simulink model "power_PSTdeltahex"  (Simulink 6.0)
settings: Solver=ode23tb  StartTime=0.0  StopTime=50  MaxStep=1/60  RelTol=1e-4  AbsTol=1e-3
undefined symbols (not defined in the file or in its folder): I21_init_imag, I21_init_real
libraries: powerlib x117, powerlib_extras x19, simulink_extras x1
(part 2 of 3)

== system power_PSTdeltahex/Three-Phase OLTC Phase Shifting Transformer Delta-Hexagonal/TransfoB ==
  OLTC : Subsystem
  Transformer : Subsystem  AncestorBlock=powerlib/Elements/Multi-Winding Transformer  mask(Multi-Windings Transformer){LeftWindings=1, RightWindings=1, TappedWindings=taps on upper right winding, NumberOfTaps=19, NominalPower=[Pnom3ph/3 Fnom], NominalVoltages=Vnom_Windings, WindingResistances=Rpu_Windings, WindingInductances=Xpu_Windings, SetSaturation=off, Rm=Rmag, Lm=Lmag, Saturation=SaturationCurrentFlux, Hysteresis=off, DataFile='hysteresis.mat', Measurements=None, InitialFlux=26.7622502223547, TransfoNumber=1}
      mask prompts: LeftWindings "Number of windings on left side"; RightWindings "Number of windings on right side"; TappedWindings "Tapped winding"; NumberOfTaps "----  Number of taps (equally spaced):"; NominalPower "Nominal power and frequency [Pn(VA) fn(Hz)]:"; NominalVoltages "Winding nominal voltages [U1 U2 ... Un] (Vrms):"; WindingResistances "Winding resistances [R1 R2 ... Rn] (pu):"; WindingInductances "Winding leakage inductances [L1 L2 ... Ln] (pu):"; SetSaturation "Saturable core"; Rm "Magnetization resistance  Rm (pu)"; Lm "Magnetization reactance Lm (pu)"; Saturation "Saturation characteristic (pu) [ i1 ,  phi1 ;  i2 , phi2 ; ... ]"; Hysteresis "Simulate hysteresis"; DataFile "----  Hysteresis Data Mat file"; InitialFlux "Initial Flux (internal use)"; TransfoNumber "Device number (internal use)"
      mask init: same as power_PSTdeltahex/Three-Phase OLTC Phase Shifting Transformer Delta-Hexagonal/TransfoA/Transformer
      mask StyleString: edit,edit,popup(no taps|taps on upper left winding|taps on upper right winding),edit,edit,edit,edit,edit,checkbox,edit,edit,edit,checkbox,edit,popup(None|Winding voltages|Winding currents|Flux and excitation current ( Imag + IRm )|Flux and magnetization current ( Imag )|All measurements (V I Flux)),edit,edit
      mask CallbackString: powericon('NWindingsTransformerCback',gcb,0);|powericon('NWindingsTransformerCback',gcb,0);|powericon('NWindingsTransformerCback',gcb,1);|powericon('NWindingsTransformerCback',gcb,1);|||||powericon('NWindingsTransformerCback',gcb,0);||||powericon('NWindingsTransformerCback',gcb,0);||||
  W2- : PMIOPort  Orientation=left  Port=1  Side=Left
  W2_tap- : PMIOPort  Orientation=left  Port=2  Side=Left
  W1- : PMIOPort  Port=3  Side=Left
  W2+ : PMIOPort  Orientation=left  Port=4  Side=Right
  W2_tap+ : PMIOPort  Orientation=left  Port=5  Side=Right
  W1+ : PMIOPort  Port=6  Side=Right
  wires:
  [SwInversion] -> OLTC/3(SwInv)
  [SwTransfer] -> OLTC/2(SwR)
  [SwSelect] -> OLTC/1(Sw0/10)
  connections:
  W2-/RConn1 -- OLTC/LConn21 -- Transformer/RConn21
  Transformer/RConn20 -- OLTC/LConn20
  Transformer/RConn19 -- OLTC/LConn19
  Transformer/RConn18 -- OLTC/LConn18
  Transformer/RConn17 -- OLTC/LConn17
  Transformer/RConn16 -- OLTC/LConn16
  Transformer/RConn15 -- OLTC/LConn15
  Transformer/RConn14 -- OLTC/LConn14
  Transformer/RConn13 -- OLTC/LConn13
  Transformer/RConn12 -- OLTC/LConn12
  Transformer/RConn11 -- OLTC/LConn11
  Transformer/RConn10 -- OLTC/LConn10
  Transformer/RConn9 -- OLTC/LConn9
  Transformer/RConn8 -- OLTC/LConn8
  Transformer/RConn7 -- OLTC/LConn7
  Transformer/RConn6 -- OLTC/LConn6
  Transformer/RConn5 -- OLTC/LConn5
  Transformer/RConn4 -- OLTC/LConn4
  Transformer/RConn3 -- OLTC/LConn3
  Transformer/RConn2 -- OLTC/LConn2
  W2+/RConn1 -- OLTC/LConn1 -- Transformer/RConn1
  OLTC/RConn2 -- W2_tap-/RConn1
  OLTC/RConn1 -- W2_tap+/RConn1
  W1+/RConn1 -- Transformer/LConn1
  W1-/RConn1 -- Transformer/LConn2

== system power_PSTdeltahex/Three-Phase OLTC Phase Shifting Transformer Delta-Hexagonal/TransfoC ==
  OLTC : Subsystem
  Transformer : Subsystem  AncestorBlock=powerlib/Elements/Multi-Winding Transformer  mask(Multi-Windings Transformer){LeftWindings=1, RightWindings=1, TappedWindings=taps on upper right winding, NumberOfTaps=19, NominalPower=[Pnom3ph/3 Fnom], NominalVoltages=Vnom_Windings, WindingResistances=Rpu_Windings, WindingInductances=Xpu_Windings, SetSaturation=off, Rm=Rmag, Lm=Lmag, Saturation=SaturationCurrentFlux, Hysteresis=off, DataFile='hysteresis.mat', Measurements=None, InitialFlux=26.7622502223547, TransfoNumber=1}
      mask prompts: LeftWindings "Number of windings on left side"; RightWindings "Number of windings on right side"; TappedWindings "Tapped winding"; NumberOfTaps "----  Number of taps (equally spaced):"; NominalPower "Nominal power and frequency [Pn(VA) fn(Hz)]:"; NominalVoltages "Winding nominal voltages [U1 U2 ... Un] (Vrms):"; WindingResistances "Winding resistances [R1 R2 ... Rn] (pu):"; WindingInductances "Winding leakage inductances [L1 L2 ... Ln] (pu):"; SetSaturation "Saturable core"; Rm "Magnetization resistance  Rm (pu)"; Lm "Magnetization reactance Lm (pu)"; Saturation "Saturation characteristic (pu) [ i1 ,  phi1 ;  i2 , phi2 ; ... ]"; Hysteresis "Simulate hysteresis"; DataFile "----  Hysteresis Data Mat file"; InitialFlux "Initial Flux (internal use)"; TransfoNumber "Device number (internal use)"
      mask init: same as power_PSTdeltahex/Three-Phase OLTC Phase Shifting Transformer Delta-Hexagonal/TransfoA/Transformer
      mask StyleString: edit,edit,popup(no taps|taps on upper left winding|taps on upper right winding),edit,edit,edit,edit,edit,checkbox,edit,edit,edit,checkbox,edit,popup(None|Winding voltages|Winding currents|Flux and excitation current ( Imag + IRm )|Flux and magnetization current ( Imag )|All measurements (V I Flux)),edit,edit
      mask CallbackString: powericon('NWindingsTransformerCback',gcb,0);|powericon('NWindingsTransformerCback',gcb,0);|powericon('NWindingsTransformerCback',gcb,1);|powericon('NWindingsTransformerCback',gcb,1);|||||powericon('NWindingsTransformerCback',gcb,0);||||powericon('NWindingsTransformerCback',gcb,0);||||
  W2- : PMIOPort  Orientation=left  Port=1  Side=Left
  W2_tap- : PMIOPort  Orientation=left  Port=2  Side=Left
  W1- : PMIOPort  Port=3  Side=Left
  W2+ : PMIOPort  Orientation=left  Port=4  Side=Right
  W2_tap+ : PMIOPort  Orientation=left  Port=5  Side=Right
  W1+ : PMIOPort  Port=6  Side=Right
  wires:
  [SwSelect] -> OLTC/1(Sw0/10)
  [SwTransfer] -> OLTC/2(SwR)
  [SwInversion] -> OLTC/3(SwInv)
  connections:
  W1-/RConn1 -- Transformer/LConn2
  W1+/RConn1 -- Transformer/LConn1
  OLTC/RConn1 -- W2_tap+/RConn1
  OLTC/RConn2 -- W2_tap-/RConn1
  Transformer/RConn1 -- OLTC/LConn1 -- W2+/RConn1
  Transformer/RConn2 -- OLTC/LConn2
  Transformer/RConn3 -- OLTC/LConn3
  Transformer/RConn4 -- OLTC/LConn4
  Transformer/RConn5 -- OLTC/LConn5
  Transformer/RConn6 -- OLTC/LConn6
  Transformer/RConn7 -- OLTC/LConn7
  Transformer/RConn8 -- OLTC/LConn8
  Transformer/RConn9 -- OLTC/LConn9
  Transformer/RConn10 -- OLTC/LConn10
  Transformer/RConn11 -- OLTC/LConn11
  Transformer/RConn12 -- OLTC/LConn12
  Transformer/RConn13 -- OLTC/LConn13
  Transformer/RConn14 -- OLTC/LConn14
  Transformer/RConn15 -- OLTC/LConn15
  Transformer/RConn16 -- OLTC/LConn16
  Transformer/RConn17 -- OLTC/LConn17
  Transformer/RConn18 -- OLTC/LConn18
  Transformer/RConn19 -- OLTC/LConn19
  Transformer/RConn20 -- OLTC/LConn20
  Transformer/RConn21 -- OLTC/LConn21 -- W2-/RConn1

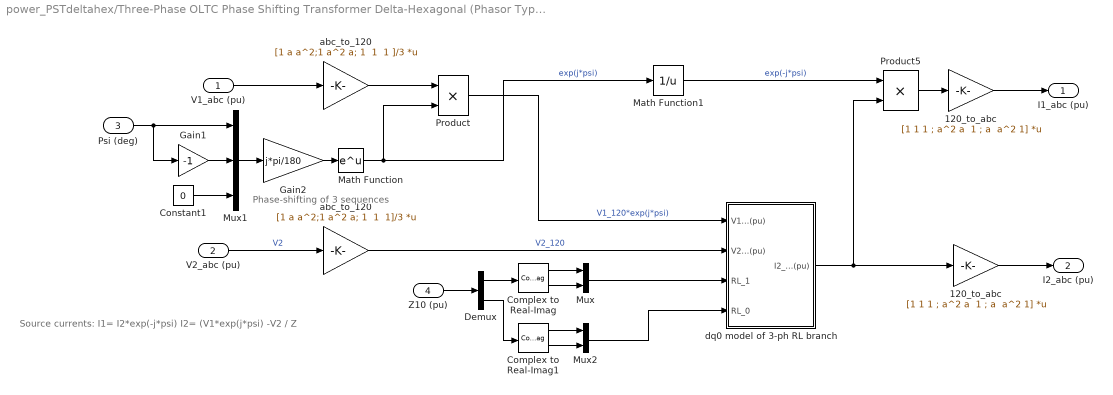
== system power_PSTdeltahex/Three-Phase OLTC Phase Shifting Transformer Delta-Hexagonal (Phasor Type)/ Currents ==
  note: Source currents:
      | I1= I2*exp(-j*psi)
      | I2= (V1*exp(j*psi) -V2 / Z
  note: Phase-shifting
      | of 3 sequences
  V1_abc (pu) : Inport  Port=1  LatchInput=off
  V2_abc (pu) : Inport  Port=2  LatchInput=off
  Psi (deg) : Inport  Port=3  LatchInput=off
  Z10 (pu) : Inport  Port=4  LatchInput=off
  120_to_abc : Gain  Gain="[1 1 1 ; a^2 a  1 ; a  a^2 1]"  Multiplication=Matrix(K*u)  SaturateOnIntegerOverflow=on
  "120_to_abc " : Gain  Gain="[1 1 1 ; a^2 a  1 ; a  a^2 1]"  Multiplication=Matrix(K*u)  SaturateOnIntegerOverflow=on
  Complex to Real-Imag : ComplexToRealImag
  Complex to Real-Imag1 : ComplexToRealImag
  Constant1 : Constant  Value=0
  Demux : Demux  Outputs=2
  Gain1 : Gain  Gain=-1  SaturateOnIntegerOverflow=on
  Gain2 : Gain  Gain=j*pi/180  SaturateOnIntegerOverflow=on
  Math Function : Math  SaturateOnIntegerOverflow=on
  Math Function1 : Math  Operator=reciprocal  SaturateOnIntegerOverflow=on
  Mux : Mux  Inputs=2
  Mux1 : Mux  Inputs=3
  Mux2 : Mux  Inputs=2
  Product : Product  SaturateOnIntegerOverflow=on
  Product5 : Product  SaturateOnIntegerOverflow=on
  abc_to_120 : Gain  Gain="[1 a a^2;1 a^2 a; 1  1  1 ]/3"  Multiplication=Matrix(K*u)  SaturateOnIntegerOverflow=on
  "abc_to_120 " : Gain  Gain="[1 a a^2;1 a^2 a; 1  1  1]/3"  Multiplication=Matrix(K*u)  SaturateOnIntegerOverflow=on
  dq0 model of 3-ph RL branch : Subsystem
  I1_abc (pu) : Outport
  "I2_abc (pu) " : Outport  Port=2
  wires:
  Gain2/1 -> Math Function/1
  Product/1 -> dq0 model of 3-ph RL branch/1(V1_120(pu))  "V1_120*exp(j*psi)"
  Math Function/1 -> Math Function1/1, Product/2  "exp(j*psi)"
  V1_abc (pu)/1 -> abc_to_120/1
  V2_abc (pu)/1 -> "abc_to_120 "/1  "V2"
  Product5/1 -> "120_to_abc "/1
  Z10 (pu)/1 -> Demux/1
  Math Function1/1 -> Product5/1  "exp(-j*psi)"
  Psi (deg)/1 -> Gain1/1, Mux1/1
  Mux1/1 -> Gain2/1
  Gain1/1 -> Mux1/2
  Constant1/1 -> Mux1/3
  dq0 model of 3-ph RL branch/1(I2_120 (pu)) -> Product5/2, 120_to_abc/1
  Demux/1 -> Complex to Real-Imag/1
  Demux/2 -> Complex to Real-Imag1/1
  Complex to Real-Imag/1 -> Mux/1
  Complex to Real-Imag/2 -> Mux/2
  Mux/1 -> dq0 model of 3-ph RL branch/3(RL_1)
  Complex to Real-Imag1/1 -> Mux2/1
  Complex to Real-Imag1/2 -> Mux2/2
  Mux2/1 -> dq0 model of 3-ph RL branch/4(RL_0)
  abc_to_120/1 -> Product/1
  "abc_to_120 "/1 -> dq0 model of 3-ph RL branch/2(V2_120(pu))  "V2_120"
  120_to_abc/1 -> "I2_abc (pu) "/1
  "120_to_abc "/1 -> I1_abc (pu)/1

== system power_PSTdeltahex/Three-Phase OLTC Phase Shifting Transformer Delta-Hexagonal (Phasor Type)/Current Source ==
  I1_abc : Inport  Orientation=left  Port=1  LatchInput=off
  I2_abc : Inport  Port=2  LatchInput=off
  Demux : Demux  Outputs=3
  Demux1 : Demux  Orientation=left  Outputs=3
  Gain2 : Gain  Gain=Ibase  SaturateOnIntegerOverflow=on
  Gain4 : Gain  Orientation=left  Gain=Ibase  SaturateOnIntegerOverflow=on
  Ground1 : powerlib/Elements/Ground  Orientation=down  PhysicalDomain=powersysdomain  SubClassName=unknown  LeftPortType=p1  RightPortType=p1  LConnTagsString=a
  Ground2 : powerlib/Elements/Ground  Orientation=down  PhysicalDomain=powersysdomain  SubClassName=unknown  LeftPortType=p1  RightPortType=p1  LConnTagsString=a
  IA : powerlib/Electrical Sources/Controlled Current Source  Initialize=on  Amplitude=I1A_init_mag  Phase=I1A_init_pha  Frequency=Fnom  Measurements=None
  IB : powerlib/Electrical Sources/Controlled Current Source  Initialize=on  Amplitude=I1B_init_mag  Phase=I1B_init_pha  Frequency=Fnom  Measurements=None
  IC : powerlib/Electrical Sources/Controlled Current Source  Initialize=on  Amplitude=I1C_init_mag  Phase=I1C_init_pha  Frequency=Fnom  Measurements=None
  Ia : powerlib/Electrical Sources/Controlled Current Source  Initialize=on  Amplitude=I2A_init_mag  Phase=I2A_init_pha  Frequency=Fnom  Measurements=None
  Ib : powerlib/Electrical Sources/Controlled Current Source  Initialize=on  Amplitude=I2B_init_mag  Phase=I2B_init_pha  Frequency=Fnom  Measurements=None
  Ic : powerlib/Electrical Sources/Controlled Current Source  Initialize=on  Amplitude=I2C_init_mag  Phase=I2C_init_pha  Frequency=Fnom  Measurements=None
  A : PMIOPort  Port=1  Side=Left
  a : PMIOPort  Orientation=left  Port=2  Side=Right
  B : PMIOPort  Port=3  Side=Left
  b : PMIOPort  Orientation=left  Port=4  Side=Right
  c : PMIOPort  Orientation=left  Port=5  Side=Right
  C : PMIOPort  Port=6  Side=Left
  wires:
  I1_abc/1 -> Gain4/1
  I2_abc/1 -> Gain2/1
  Demux/3 -> Ic/1
  Demux/2 -> Ib/1
  Demux/1 -> Ia/1
  Demux1/3 -> IC/1
  Demux1/2 -> IB/1
  Demux1/1 -> IA/1
  Gain2/1 -> Demux/1
  Gain4/1 -> Demux1/1
  connections:
  Ic/RConn1 -- c/RConn1
  Ib/RConn1 -- b/RConn1
  Ia/RConn1 -- a/RConn1
  C/RConn1 -- IC/LConn1
  B/RConn1 -- IB/LConn1
  A/RConn1 -- IA/LConn1
  Ib/LConn1 -- Ia/LConn1 -- Ic/LConn1 -- Ground1/LConn1
  IB/RConn1 -- IA/RConn1 -- IC/RConn1 -- Ground2/LConn1

== system power_PSTdeltahex/Three-Phase OLTC Phase Shifting Transformer Delta-Hexagonal (Phasor Type)/Subsystem ==
  note: Delta Hexagonal Phase Shifting Transformer
  note: Each phase consists of two windings ( winding W1(no taps)  and tapped winding W2)
      | Voltage ratio= 1:1  Rated voltage of each winding=2/3*(VnomPh-Ph)
      | Two OLTCs connected to inputs (ABC) and outputs (abc)
      | select taps symmetrical with respect to center of tapped windings W2
  note: A        a
      |                  |        |
      |              A A A A A A A A A A
      |            B          W2         C
      |          B                         C
      |        B    W1                  W1   C
      |      B                                 C
      |    B                                     C
      |  +                                         +
      |    C                                     B
      | c--->C                                 B<---B
      |        C    W2                  W2   B
      |     C--->C                         B<---b
      |            C          W1         B
      |              A A A A A A A A A A
  note: k=relative tap position
      |     k=Tap/NumberOfTaps  (-1<= k <= 1 )
      |
      | Psi= Phase shift  of output voltage (abc)  with respect to input voltage (ABC)
      | Psi varies from +60 deg. to -60 deg. when k varies from -1 to +1
      | Psi= 2*atan(-k/sqrt(3)
      |
      | Positive- and zero-sequence impedances vary with tap position k
  note: Positive sequence impedance:
      |  Z1 = Z1@ maximum_tap * kz1
      |           where :
      | kz1 =k/(2*(k^2+3))*(-3*k^2  +2k  +9)
      |   k  =  relative tap position (  0 <= k <=1 )
      |
      | Zero sequence impedance:
      |  Z0 = Zm*k^2

== system power_PSTdeltahex/Three-Phase OLTC Phase Shifting Transformer Delta-Hexagonal (Phasor Type)/Tap Changer Control ==
  Up : Inport  Port=1  LatchInput=off
  Down : Inport  Port=2  LatchInput=off
  Constant : Constant  Value=-1
  Constant1 : Constant
  Determine tap positon : Subsystem
  Edge Detector : powerlib_extras/Control  Blocks/Edge Detector  model=Rising  ic=0
  Logical Operator : Logic  Operator=OR  AllPortsSameDT=off
  Logical Operator1 : Logic  AllPortsSameDT=off
  Mechanical Delay : TransportDelay  DelayTime=MecDelay  InitialInput=InitialPosition
  Memory : Memory  Orientation=left  X0=1  InheritSampleTime=on
  Relational Operator : RelationalOperator  Operator===  LogicOutDataTypeMode=Specify via dialog  LogicDataType=float('double')
  Switch : Switch  Threshold=0.5  SaturateOnIntegerOverflow=on
  TapNo : Outport
  Ready : Outport  Port=2
  wires:
  Mechanical Delay/1 -> TapNo/1, Relational Operator/2
  Logical Operator1/1 -> Determine tap positon/Trigger
  Up/1 -> Logical Operator/1
  Down/1 -> Logical Operator/2, Switch/2
  Constant/1 -> Switch/1
  Constant1/1 -> Switch/3
  Switch/1 -> Determine tap positon/1(NewTap)
  Determine tap positon/1(TapNo) -> Mechanical Delay/1, Relational Operator/1
  Relational Operator/1 -> Memory/1
  Memory/1 -> Logical Operator1/1, Ready/1
  Logical Operator/1 -> Edge Detector/1
  Edge Detector/1 -> Logical Operator1/2

== system power_PSTdeltahex/Three-Phase OLTC Phase Shifting Transformer Delta-Hexagonal (Phasor Type)/Z1 Z0 impedances Computation  ==
  note: Positive sequence impedance:
      |  Z1 = Z1@ maximum_tap * kz1
      |           where :
      | kz1 =k/(2*(k^2+3))*(-3*k^2  +2k +9)
      |   k  =  relative tap position (  0 <= k <=1 )
      |
      | Zero sequence impedance:
      |  Z0 = Zm*k^2
  k : Inport  Port=1  LatchInput=off
  Z1maxpu : Inport  Port=2  LatchInput=off
  Zmpu : Inport  Port=3  LatchInput=off
  Abs : Abs  ZeroCross=off  SaturateOnIntegerOverflow=on
  Gain1 : Gain  Gain=2  SaturateOnIntegerOverflow=on
  Gain2 : Gain  Gain=3  SaturateOnIntegerOverflow=on
  Gain3 : Gain  Gain=2  SaturateOnIntegerOverflow=on
  Math Function2 : Math  Orientation=down  Operator=square  SaturateOnIntegerOverflow=on
  Mux : Mux  Inputs=2
  Product1 : Product  Inputs=*/*  SaturateOnIntegerOverflow=on
  Product5 : Product  Inputs=**  SaturateOnIntegerOverflow=on
  Product6 : Product  Inputs=**  SaturateOnIntegerOverflow=on
  Sum : Sum  SaturateOnIntegerOverflow=on
  Sum1 : Sum  Inputs=++-  SaturateOnIntegerOverflow=on
  psi4 : Constant  Value=3
  psi5 : Constant  Value=9
  Z10 : Outport
  wires:
  Product5/1 -> Mux/2  "Z0"
  Abs/1 -> Math Function2/1, Product1/1, Gain1/1  "k"
  k/1 -> Abs/1
  Mux/1 -> Z10/1
  Product6/1 -> Mux/1  "Z1"
  Product1/1 -> Product6/2  "kz1"
  Z1maxpu/1 -> Product6/1
  Zmpu/1 -> Product5/2
  Sum1/1 -> Product1/3  "-3*k^2 +2*k +9"
  psi5/1 -> Sum1/1
  psi4/1 -> Sum/2
  Sum/1 -> Gain3/1
  Math Function2/1 -> Sum/1, Product5/1, Gain2/1
  Gain1/1 -> Sum1/2
  Gain2/1 -> Sum1/3
  Gain3/1 -> Product1/2  "2*(k^2+3)"

== system power_PSTdeltahex/Three-Phase OLTC Phase Shifting Transformer Delta-Hexagonal (Phasor Type)/Zmin Saturation ==
  In1 : Inport  Port=1  LatchInput=off
  Complex to Real-Imag : ComplexToRealImag
  Real-Imag to Complex : RealImagToComplex
  Saturation2 : Saturate  UpperLimit=1000  LowerLimit=1e-3
  Saturation3 : Saturate  UpperLimit=1000  LowerLimit=1e-3
  Out1 : Outport
  wires:
  In1/1 -> Complex to Real-Imag/1
  Real-Imag to Complex/1 -> Out1/1
  Saturation3/1 -> Real-Imag to Complex/2
  Complex to Real-Imag/2 -> Saturation3/1
  Saturation2/1 -> Real-Imag to Complex/1
  Complex to Real-Imag/1 -> Saturation2/1

== system power_PSTdeltahex/Three-Phase OLTC Phase Shifting Transformer Delta-Hexagonal/OLTC Control/Monostable ==
  note: Monostable
  note: Silvano Casoria
      | Power System Simulation Laboratory
      | IREQ, Hydro-Quebec
  In : Inport  Port=1  LatchInput=off
  Clock : Clock
      settings: Decimation=10
  Edge Detector : Subsystem  mask(Edge Detector){model=EdgeDetect, ic=ic}
      mask prompts: model "Edge:"; ic "Input at t = -eps:"
      mask help:
      | This block compares its present input to its previous input.
      |
      | If the input  is a logic signal (TRUE (1) or FALSE (0), the output is a one-step boolean signal TRUE  when  the specified edge (Rising, Falling or Either)  is detected.
      |
      | This block can also be used to detect the slope polarity of a continuous signal. For example, if the specified edge is  "Rising", the output is TRUE as long as the slope of the input signal is positive.
      |
      | The input value at time preceeding t=0 is specified by the parameter "Input at t=-eps"
      mask init:
      | if model~=3,
      | 	x1 = (model -1)*20;
      |     x2 = (model -1)*60;
      | 	X1=[5,20,20,35]+25; Y1=[20+x2,20+x2,80-x2,80-x2];
      | 	X2=[5,20,35]+25;    Y2=[40+x1,60-x1,40+x1];
      | 	X3=[];X4=[];Y3=[];Y4=[];
      | else
      | 	x1 = 20;
      | 	x2 = 60;
      | 	X1=[5,20,20,35]+8; Y1=[20,20,80,80];
      | 	X2=[5,20,35]+8;    Y2=[40,60,40];
      | 	X3=[5,20,20,35]+53; Y3=[20+x2,20+x2,80-x2,80-x2];
      | 	X4=[5,20,35]+53;    Y4=[40+x1,60-x1,40+x1];
      | end
      mask Display: plot(0,0,100,100, X1,Y1,X2,Y2,X3,Y3,X4,Y4);
  Logical Operator1 : Logic
  Logical Operator2 : Logic  Orientation=left  Operator=NOT  Inputs=1
  Memory : Memory  Orientation=left  InheritSampleTime=on
  Relational Operator : RelationalOperator  Operator=>  InputSameDT=on
  Sample & Hold : powerlib_extras/Control  Blocks/Sample & Hold  ic=-1e6
  Sum : Sum  SaturateOnIntegerOverflow=on  InputSameDT=on
  T_monostable : Constant  Value=t_mono - eps
  Out : Outport
  wires:
  In/1 -> Edge Detector/1(In)
  Relational Operator/1 -> Out/1, Memory/1
  Logical Operator2/1 -> Logical Operator1/1
  Edge Detector/1(Out) -> Logical Operator1/2
  Memory/1 -> Logical Operator2/1
  Sample & Hold/1 -> Sum/1
  Sum/1 -> Relational Operator/1
  Clock/1 -> Relational Operator/2, Sample & Hold/1
  T_monostable/1 -> Sum/2
  Logical Operator1/1 -> Sample & Hold/2

== system power_PSTdeltahex/Three-Phase OLTC Phase Shifting Transformer Delta-Hexagonal/OLTC Control/Set Reset ==
  Tap : Inport  Port=1  LatchInput=off
  Constant1 : Constant  Value=-1
  Constant2 : Constant
  Edge Detector1 : powerlib_extras/Control  Blocks/Edge Detector  model=Rising  ic=0
  Edge Detector2 : powerlib_extras/Control  Blocks/Edge Detector  model=Falling  ic=0
  Logical Operator1 : Logic  AllPortsSameDT=off
  Logical Operator2 : Logic  AllPortsSameDT=off
  Relational Operator1 : RelationalOperator  Operator===
  Relational Operator2 : RelationalOperator  Operator===
  Set : Outport
  Reset : Outport  Port=2
  wires:
  Logical Operator1/1 -> Set/1
  Edge Detector1/1 -> Logical Operator1/1
  Relational Operator2/1 -> Logical Operator1/2
  Constant2/1 -> Relational Operator2/2
  Tap/1 -> Relational Operator2/1, Edge Detector1/1, Relational Operator1/1, Edge Detector2/1
  Logical Operator2/1 -> Reset/1
  Edge Detector2/1 -> Logical Operator2/1
  Relational Operator1/1 -> Logical Operator2/2
  Constant1/1 -> Relational Operator1/2

== system power_PSTdeltahex/Three-Phase OLTC Phase Shifting Transformer Delta-Hexagonal/OLTC Control/Tap Changer Control ==
  Up : Inport  Port=1  LatchInput=off
  Down : Inport  Port=2  LatchInput=off
  Constant : Constant  Value=-1
  Constant1 : Constant
  Determine tap positon : Subsystem
  Edge Detector : powerlib_extras/Control  Blocks/Edge Detector  model=Rising  ic=0
  Logical Operator : Logic  Operator=OR  AllPortsSameDT=off
  Logical Operator1 : Logic  AllPortsSameDT=off
  Mechanical Delay : TransportDelay  DelayTime=MecDelay  InitialInput=InitialPosition
  Memory : Memory  Orientation=left  X0=1  InheritSampleTime=on
  Relational Operator : RelationalOperator  Operator===  LogicOutDataTypeMode=Specify via dialog  LogicDataType=float('double')
  Switch : Switch  Threshold=0.5  SaturateOnIntegerOverflow=on
  TapNo : Outport
  Ready : Outport  Port=2
  wires:
  Edge Detector/1 -> Logical Operator1/2
  Logical Operator/1 -> Edge Detector/1
  Memory/1 -> Ready/1, Logical Operator1/1
  Relational Operator/1 -> Memory/1
  Determine tap positon/1(TapNo) -> Relational Operator/1, Mechanical Delay/1
  Switch/1 -> Determine tap positon/1(NewTap)
  Constant1/1 -> Switch/3
  Constant/1 -> Switch/1
  Down/1 -> Switch/2, Logical Operator/2
  Up/1 -> Logical Operator/1
  Logical Operator1/1 -> Determine tap positon/Trigger
  Mechanical Delay/1 -> Relational Operator/2, TapNo/1

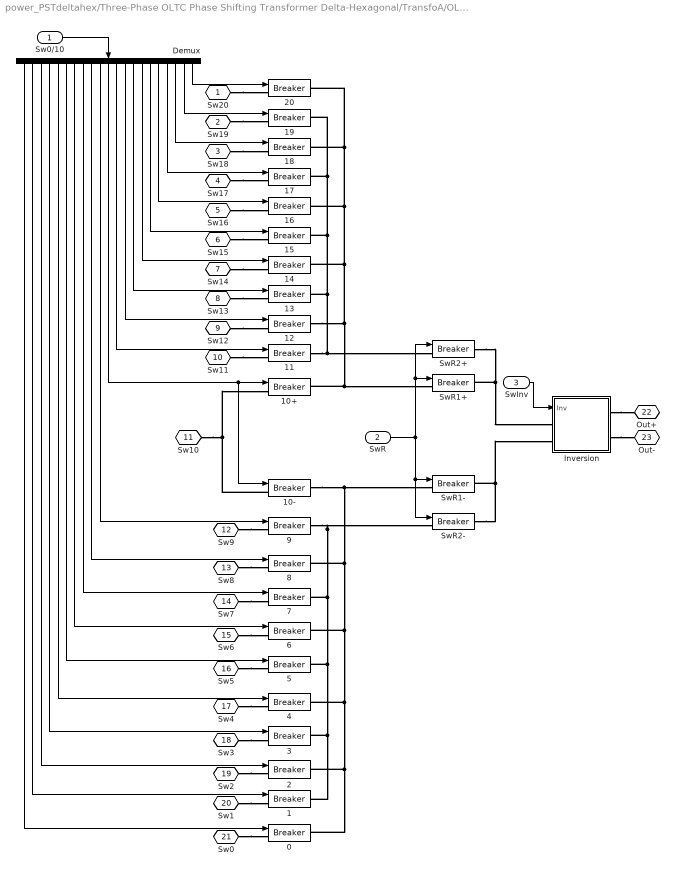
== system power_PSTdeltahex/Three-Phase OLTC Phase Shifting Transformer Delta-Hexagonal/TransfoA/OLTC ==
  Sw0/10 : Inport  Port=1  LatchInput=off
  SwR : Inport  Port=2  LatchInput=off
  SwInv : Inport  Port=3  LatchInput=off
  "0  " : powerlib/Elements/Breaker  BreakerResistance=Ron  InitialState=InitialStates(1)  SnubberResistance=Rsnub  SnubberCapacitance=inf  SwitchingTimes="[ 1/60  5/60 ]"  External=on  Measurements=None
  "1  " : powerlib/Elements/Breaker  BreakerResistance=Ron  InitialState=InitialStates(2)  SnubberResistance=Rsnub  SnubberCapacitance=inf  SwitchingTimes="[ 1/60  5/60 ]"  External=on  Measurements=None
  "10+  " : powerlib/Elements/Breaker  BreakerResistance=Ron  InitialState=InitialStates(11)  SnubberResistance=1e6  SnubberCapacitance=Rsnub  SwitchingTimes="[ 1/60  5/60 ]"  External=on  Measurements=None
  10- : powerlib/Elements/Breaker  BreakerResistance=Ron  InitialState=InitialStates(11)  SnubberResistance=Rsnub  SnubberCapacitance=inf  SwitchingTimes="[ 1/60  5/60 ]"  External=on  Measurements=None
  11 : powerlib/Elements/Breaker  BreakerResistance=Ron  InitialState=InitialStates(12)  SnubberResistance=Rsnub  SnubberCapacitance=inf  SwitchingTimes="[ 1/60  5/60 ]"  External=on  Measurements=None
  12 : powerlib/Elements/Breaker  BreakerResistance=Ron  InitialState=InitialStates(13)  SnubberResistance=Rsnub  SnubberCapacitance=inf  SwitchingTimes="[ 1/60  5/60 ]"  External=on  Measurements=None
  13 : powerlib/Elements/Breaker  BreakerResistance=Ron  InitialState=InitialStates(14)  SnubberResistance=Rsnub  SnubberCapacitance=inf  SwitchingTimes="[ 1/60  5/60 ]"  External=on  Measurements=None
  14 : powerlib/Elements/Breaker  BreakerResistance=Ron  InitialState=InitialStates(15)  SnubberResistance=Rsnub  SnubberCapacitance=inf  SwitchingTimes="[ 1/60  5/60 ]"  External=on  Measurements=None
  15 : powerlib/Elements/Breaker  BreakerResistance=Ron  InitialState=InitialStates(16)  SnubberResistance=Rsnub  SnubberCapacitance=inf  SwitchingTimes="[ 1/60  5/60 ]"  External=on  Measurements=None
  "16  " : powerlib/Elements/Breaker  BreakerResistance=Ron  InitialState=InitialStates(17)  SnubberResistance=Rsnub  SnubberCapacitance=inf  SwitchingTimes="[ 1/60  5/60 ]"  External=on  Measurements=None
  17 : powerlib/Elements/Breaker  BreakerResistance=Ron  InitialState=InitialStates(18)  SnubberResistance=Rsnub  SnubberCapacitance=inf  SwitchingTimes="[ 1/60  5/60 ]"  External=on  Measurements=None
  18 : powerlib/Elements/Breaker  BreakerResistance=Ron  InitialState=InitialStates(19)  SnubberResistance=Rsnub  SnubberCapacitance=inf  SwitchingTimes="[ 1/60  5/60 ]"  External=on  Measurements=None
  19 : powerlib/Elements/Breaker  BreakerResistance=Ron  InitialState=InitialStates(20)  SnubberResistance=Rsnub  SnubberCapacitance=inf  SwitchingTimes="[ 1/60  5/60 ]"  External=on  Measurements=None
  "2    " : powerlib/Elements/Breaker  BreakerResistance=Ron  InitialState=InitialStates(3)  SnubberResistance=Rsnub  SnubberCapacitance=inf  SwitchingTimes="[ 1/60  5/60 ]"  External=on  Measurements=None
  20 : powerlib/Elements/Breaker  BreakerResistance=Ron  InitialState=InitialStates(21)  SnubberResistance=Rsnub  SnubberCapacitance=inf  SwitchingTimes="[ 1/60  5/60 ]"  External=on  Measurements=None
  "3  " : powerlib/Elements/Breaker  BreakerResistance=Ron  InitialState=InitialStates(4)  SnubberResistance=Rsnub  SnubberCapacitance=inf  SwitchingTimes="[ 1/60  5/60 ]"  External=on  Measurements=None
  "4  " : powerlib/Elements/Breaker  BreakerResistance=Ron  InitialState=InitialStates(5)  SnubberResistance=Rsnub  SnubberCapacitance=inf  SwitchingTimes="[ 1/60  5/60 ]"  External=on  Measurements=None
  5 : powerlib/Elements/Breaker  BreakerResistance=Ron  InitialState=InitialStates(6)  SnubberResistance=Rsnub  SnubberCapacitance=inf  SwitchingTimes="[ 1/60  5/60 ]"  External=on  Measurements=None
  6 : powerlib/Elements/Breaker  BreakerResistance=Ron  InitialState=InitialStates(7)  SnubberResistance=Rsnub  SnubberCapacitance=inf  SwitchingTimes="[ 1/60  5/60 ]"  External=on  Measurements=None
  7 : powerlib/Elements/Breaker  BreakerResistance=Ron  InitialState=InitialStates(8)  SnubberResistance=Rsnub  SnubberCapacitance=inf  SwitchingTimes="[ 1/60  5/60 ]"  External=on  Measurements=None
  8 : powerlib/Elements/Breaker  BreakerResistance=Ron  InitialState=InitialStates(9)  SnubberResistance=Rsnub  SnubberCapacitance=inf  SwitchingTimes="[ 1/60  5/60 ]"  External=on  Measurements=None
  9 : powerlib/Elements/Breaker  BreakerResistance=Ron  InitialState=InitialStates(10)  SnubberResistance=Rsnub  SnubberCapacitance=inf  SwitchingTimes="[ 1/60  5/60 ]"  External=on  Measurements=None
  Demux : Demux  Orientation=down  Outputs=21
  Inversion : Subsystem
  SwR1+ : powerlib/Elements/Breaker  BreakerResistance=Ron  InitialState=1  SnubberResistance=R  SnubberCapacitance=inf  SwitchingTimes="[ 1/60  5/60 ]"  External=on  Measurements=None
  SwR1- : powerlib/Elements/Breaker  BreakerResistance=Ron  InitialState=1  SnubberResistance=R  SnubberCapacitance=inf  SwitchingTimes="[ 1/60  5/60 ]"  External=on  Measurements=None
  SwR2+ : powerlib/Elements/Breaker  BreakerResistance=Ron  InitialState=1  SnubberResistance=R  SnubberCapacitance=inf  SwitchingTimes="[ 1/60  5/60 ]"  External=on  Measurements=None
  SwR2- : powerlib/Elements/Breaker  BreakerResistance=Ron  InitialState=1  SnubberResistance=R  SnubberCapacitance=inf  SwitchingTimes="[ 1/60  5/60 ]"  External=on  Measurements=None
  Sw20 : PMIOPort  Port=1  Side=Left
  Sw19 : PMIOPort  Port=2  Side=Left
  Sw18 : PMIOPort  Port=3  Side=Left
  Sw17 : PMIOPort  Port=4  Side=Left
  Sw16 : PMIOPort  Port=5  Side=Left
  Sw15 : PMIOPort  Port=6  Side=Left
  Sw14 : PMIOPort  Port=7  Side=Left
  Sw13 : PMIOPort  Port=8  Side=Left
  Sw12 : PMIOPort  Port=9  Side=Left
  Sw11 : PMIOPort  Port=10  Side=Left
  Sw10 : PMIOPort  Port=11  Side=Left
  "Sw9 " : PMIOPort  Port=12  Side=Left
  Sw8 : PMIOPort  Port=13  Side=Left
  Sw7 : PMIOPort  Port=14  Side=Left
  Sw6 : PMIOPort  Port=15  Side=Left
  Sw5 : PMIOPort  Port=16  Side=Left
  Sw4 : PMIOPort  Port=17  Side=Left
  Sw3 : PMIOPort  Port=18  Side=Left
  "Sw2 " : PMIOPort  Port=19  Side=Left
  Sw1 : PMIOPort  Port=20  Side=Left
  Sw0 : PMIOPort  Port=21  Side=Left
  Out+ : PMIOPort  Orientation=left  Port=22  Side=Right
  Out- : PMIOPort  Orientation=left  Port=23  Side=Right
  wires:
  Sw0/10/1 -> Demux/1
  Demux/1 -> "0  "/1
  Demux/2 -> "1  "/1
  Demux/3 -> "2    "/1
  Demux/4 -> "3  "/1
  Demux/5 -> "4  "/1
  SwInv/1 -> Inversion/1(Inv)
  Demux/21 -> 20/1
  Demux/20 -> 19/1
  Demux/19 -> 18/1
  Demux/18 -> 17/1
  Demux/17 -> "16  "/1
  Demux/16 -> 15/1
  Demux/15 -> 14/1
  Demux/14 -> 13/1
  Demux/13 -> 12/1
  Demux/12 -> 11/1
  Demux/11 -> "10+  "/1, 10-/1
  Demux/10 -> 9/1
  Demux/9 -> 8/1
  Demux/8 -> 7/1
  Demux/7 -> 6/1
  Demux/6 -> 5/1
  SwR/1 -> SwR2+/1, SwR1+/1, SwR1-/1, SwR2-/1
  connections:
  Sw20/RConn1 -- 20/LConn1
  Sw19/RConn1 -- 19/LConn1
  Sw18/RConn1 -- 18/LConn1
  Sw17/RConn1 -- 17/LConn1
  Sw16/RConn1 -- "16  "/LConn1
  Sw4/RConn1 -- "4  "/LConn1
  Sw3/RConn1 -- "3  "/LConn1
  "Sw2 "/RConn1 -- "2    "/LConn1
  Sw1/RConn1 -- "1  "/LConn1
  Sw0/RConn1 -- "0  "/LConn1
  Inversion/RConn1 -- Out+/RConn1
  Inversion/RConn2 -- Out-/RConn1
  Sw5/RConn1 -- 5/LConn1
  Sw6/RConn1 -- 6/LConn1
  Sw7/RConn1 -- 7/LConn1
  Sw8/RConn1 -- 8/LConn1
  "Sw9 "/RConn1 -- 9/LConn1
  Sw15/RConn1 -- 15/LConn1
  Sw14/RConn1 -- 14/LConn1
  Sw13/RConn1 -- 13/LConn1
  Sw12/RConn1 -- 12/LConn1
  Sw11/RConn1 -- 11/LConn1
  SwR2-/RConn1 -- SwR1-/RConn1 -- Inversion/LConn2
  10-/RConn1 -- 8/RConn1 -- 6/RConn1 -- "4  "/RConn1 -- "2    "/RConn1 -- "0  "/RConn1 -- SwR1-/LConn1
  9/RConn1 -- 7/RConn1 -- 5/RConn1 -- "3  "/RConn1 -- "1  "/RConn1 -- SwR2-/LConn1
  12/RConn1 -- 14/RConn1 -- "16  "/RConn1 -- 18/RConn1 -- 20/RConn1 -- "10+  "/RConn1 -- SwR1+/LConn1
  11/RConn1 -- 13/RConn1 -- 15/RConn1 -- 17/RConn1 -- 19/RConn1 -- SwR2+/LConn1
  10-/LConn1 -- "10+  "/LConn1 -- Sw10/RConn1
  SwR2+/RConn1 -- SwR1+/RConn1 -- Inversion/LConn1

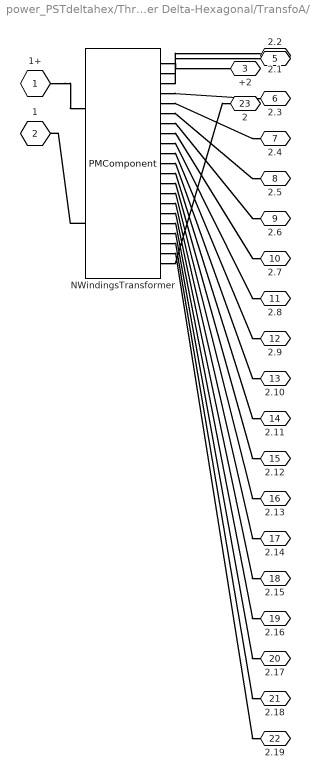
== system power_PSTdeltahex/Three-Phase OLTC Phase Shifting Transformer Delta-Hexagonal/TransfoA/Transformer ==
  NWindingsTransformer : PMComponent  PhysicalDomain=powersysdomain  LeftPortType=p1  RightPortType=p1  LConnTagsString=1|2  RConnTagsString=1|2|3|4|5|6|7|8|9|10|11|12|13|14|15|16|17|18|19|20|21
      mask Type: InnerPowersysBlock
  1+ : PMIOPort  Port=1  Side=Left
  1 : PMIOPort  Port=2  Side=Left
  +2 : PMIOPort  Orientation=left  Port=3  Side=Right
  2.1 : PMIOPort  Orientation=left  Port=4  Side=Right
  2.2 : PMIOPort  Orientation=left  Port=5  Side=Right
  2.3 : PMIOPort  Orientation=left  Port=6  Side=Right
  2.4 : PMIOPort  Orientation=left  Port=7  Side=Right
  2.5 : PMIOPort  Orientation=left  Port=8  Side=Right
  2.6 : PMIOPort  Orientation=left  Port=9  Side=Right
  2.7 : PMIOPort  Orientation=left  Port=10  Side=Right
  2.8 : PMIOPort  Orientation=left  Port=11  Side=Right
  2.9 : PMIOPort  Orientation=left  Port=12  Side=Right
  2.10 : PMIOPort  Orientation=left  Port=13  Side=Right
  2.11 : PMIOPort  Orientation=left  Port=14  Side=Right
  2.12 : PMIOPort  Orientation=left  Port=15  Side=Right
  2.13 : PMIOPort  Orientation=left  Port=16  Side=Right
  2.14 : PMIOPort  Orientation=left  Port=17  Side=Right
  2.15 : PMIOPort  Orientation=left  Port=18  Side=Right
  2.16 : PMIOPort  Orientation=left  Port=19  Side=Right
  2.17 : PMIOPort  Orientation=left  Port=20  Side=Right
  2.18 : PMIOPort  Orientation=left  Port=21  Side=Right
  2.19 : PMIOPort  Orientation=left  Port=22  Side=Right
  2 : PMIOPort  Orientation=left  Port=23  Side=Right
  connections:
  NWindingsTransformer/RConn1 -- +2/RConn1
  1+/RConn1 -- NWindingsTransformer/LConn1
  NWindingsTransformer/LConn2 -- 1/RConn1
  NWindingsTransformer/RConn2 -- 2.1/RConn1
  NWindingsTransformer/RConn3 -- 2.2/RConn1
  NWindingsTransformer/RConn4 -- 2.3/RConn1
  NWindingsTransformer/RConn5 -- 2.4/RConn1
  NWindingsTransformer/RConn6 -- 2.5/RConn1
  NWindingsTransformer/RConn7 -- 2.6/RConn1
  NWindingsTransformer/RConn8 -- 2.7/RConn1
  NWindingsTransformer/RConn9 -- 2.8/RConn1
  NWindingsTransformer/RConn10 -- 2.9/RConn1
  NWindingsTransformer/RConn21 -- 2/RConn1
  NWindingsTransformer/RConn11 -- 2.10/RConn1
  NWindingsTransformer/RConn12 -- 2.11/RConn1
  NWindingsTransformer/RConn13 -- 2.12/RConn1
  NWindingsTransformer/RConn14 -- 2.13/RConn1
  NWindingsTransformer/RConn15 -- 2.14/RConn1
  NWindingsTransformer/RConn16 -- 2.15/RConn1
  NWindingsTransformer/RConn17 -- 2.16/RConn1
  NWindingsTransformer/RConn18 -- 2.17/RConn1
  NWindingsTransformer/RConn19 -- 2.18/RConn1
  NWindingsTransformer/RConn20 -- 2.19/RConn1

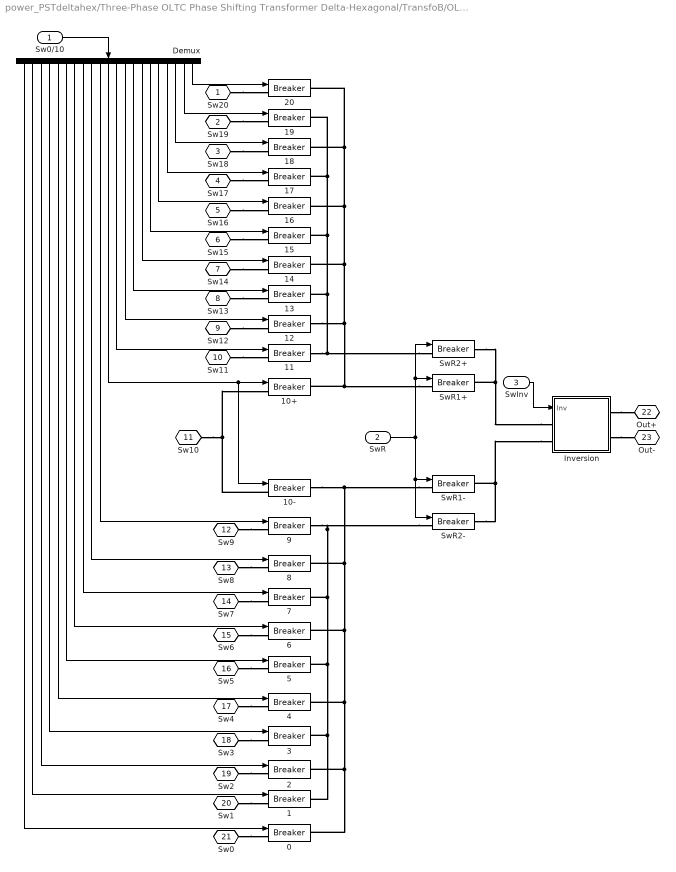
== system power_PSTdeltahex/Three-Phase OLTC Phase Shifting Transformer Delta-Hexagonal/TransfoB/OLTC ==
  Sw0/10 : Inport  Port=1  LatchInput=off
  SwR : Inport  Port=2  LatchInput=off
  SwInv : Inport  Port=3  LatchInput=off
  "0  " : powerlib/Elements/Breaker  BreakerResistance=Ron  InitialState=InitialStates(1)  SnubberResistance=Rsnub  SnubberCapacitance=inf  SwitchingTimes="[ 1/60  5/60 ]"  External=on  Measurements=None
  "1  " : powerlib/Elements/Breaker  BreakerResistance=Ron  InitialState=InitialStates(2)  SnubberResistance=Rsnub  SnubberCapacitance=inf  SwitchingTimes="[ 1/60  5/60 ]"  External=on  Measurements=None
  "10+  " : powerlib/Elements/Breaker  BreakerResistance=Ron  InitialState=InitialStates(11)  SnubberResistance=1e6  SnubberCapacitance=Rsnub  SwitchingTimes="[ 1/60  5/60 ]"  External=on  Measurements=None
  10- : powerlib/Elements/Breaker  BreakerResistance=Ron  InitialState=InitialStates(11)  SnubberResistance=Rsnub  SnubberCapacitance=inf  SwitchingTimes="[ 1/60  5/60 ]"  External=on  Measurements=None
  11 : powerlib/Elements/Breaker  BreakerResistance=Ron  InitialState=InitialStates(12)  SnubberResistance=Rsnub  SnubberCapacitance=inf  SwitchingTimes="[ 1/60  5/60 ]"  External=on  Measurements=None
  12 : powerlib/Elements/Breaker  BreakerResistance=Ron  InitialState=InitialStates(13)  SnubberResistance=Rsnub  SnubberCapacitance=inf  SwitchingTimes="[ 1/60  5/60 ]"  External=on  Measurements=None
  13 : powerlib/Elements/Breaker  BreakerResistance=Ron  InitialState=InitialStates(14)  SnubberResistance=Rsnub  SnubberCapacitance=inf  SwitchingTimes="[ 1/60  5/60 ]"  External=on  Measurements=None
  14 : powerlib/Elements/Breaker  BreakerResistance=Ron  InitialState=InitialStates(15)  SnubberResistance=Rsnub  SnubberCapacitance=inf  SwitchingTimes="[ 1/60  5/60 ]"  External=on  Measurements=None
  15 : powerlib/Elements/Breaker  BreakerResistance=Ron  InitialState=InitialStates(16)  SnubberResistance=Rsnub  SnubberCapacitance=inf  SwitchingTimes="[ 1/60  5/60 ]"  External=on  Measurements=None
  "16  " : powerlib/Elements/Breaker  BreakerResistance=Ron  InitialState=InitialStates(17)  SnubberResistance=Rsnub  SnubberCapacitance=inf  SwitchingTimes="[ 1/60  5/60 ]"  External=on  Measurements=None
  17 : powerlib/Elements/Breaker  BreakerResistance=Ron  InitialState=InitialStates(18)  SnubberResistance=Rsnub  SnubberCapacitance=inf  SwitchingTimes="[ 1/60  5/60 ]"  External=on  Measurements=None
  18 : powerlib/Elements/Breaker  BreakerResistance=Ron  InitialState=InitialStates(19)  SnubberResistance=Rsnub  SnubberCapacitance=inf  SwitchingTimes="[ 1/60  5/60 ]"  External=on  Measurements=None
  19 : powerlib/Elements/Breaker  BreakerResistance=Ron  InitialState=InitialStates(20)  SnubberResistance=Rsnub  SnubberCapacitance=inf  SwitchingTimes="[ 1/60  5/60 ]"  External=on  Measurements=None
  "2    " : powerlib/Elements/Breaker  BreakerResistance=Ron  InitialState=InitialStates(3)  SnubberResistance=Rsnub  SnubberCapacitance=inf  SwitchingTimes="[ 1/60  5/60 ]"  External=on  Measurements=None
  20 : powerlib/Elements/Breaker  BreakerResistance=Ron  InitialState=InitialStates(21)  SnubberResistance=Rsnub  SnubberCapacitance=inf  SwitchingTimes="[ 1/60  5/60 ]"  External=on  Measurements=None
  "3  " : powerlib/Elements/Breaker  BreakerResistance=Ron  InitialState=InitialStates(4)  SnubberResistance=Rsnub  SnubberCapacitance=inf  SwitchingTimes="[ 1/60  5/60 ]"  External=on  Measurements=None
  "4  " : powerlib/Elements/Breaker  BreakerResistance=Ron  InitialState=InitialStates(5)  SnubberResistance=Rsnub  SnubberCapacitance=inf  SwitchingTimes="[ 1/60  5/60 ]"  External=on  Measurements=None
  5 : powerlib/Elements/Breaker  BreakerResistance=Ron  InitialState=InitialStates(6)  SnubberResistance=Rsnub  SnubberCapacitance=inf  SwitchingTimes="[ 1/60  5/60 ]"  External=on  Measurements=None
  6 : powerlib/Elements/Breaker  BreakerResistance=Ron  InitialState=InitialStates(7)  SnubberResistance=Rsnub  SnubberCapacitance=inf  SwitchingTimes="[ 1/60  5/60 ]"  External=on  Measurements=None
  7 : powerlib/Elements/Breaker  BreakerResistance=Ron  InitialState=InitialStates(8)  SnubberResistance=Rsnub  SnubberCapacitance=inf  SwitchingTimes="[ 1/60  5/60 ]"  External=on  Measurements=None
  8 : powerlib/Elements/Breaker  BreakerResistance=Ron  InitialState=InitialStates(9)  SnubberResistance=Rsnub  SnubberCapacitance=inf  SwitchingTimes="[ 1/60  5/60 ]"  External=on  Measurements=None
  9 : powerlib/Elements/Breaker  BreakerResistance=Ron  InitialState=InitialStates(10)  SnubberResistance=Rsnub  SnubberCapacitance=inf  SwitchingTimes="[ 1/60  5/60 ]"  External=on  Measurements=None
  Demux : Demux  Orientation=down  Outputs=21
  Inversion : Subsystem
  SwR1+ : powerlib/Elements/Breaker  BreakerResistance=Ron  InitialState=1  SnubberResistance=R  SnubberCapacitance=inf  SwitchingTimes="[ 1/60  5/60 ]"  External=on  Measurements=None
  SwR1- : powerlib/Elements/Breaker  BreakerResistance=Ron  InitialState=1  SnubberResistance=R  SnubberCapacitance=inf  SwitchingTimes="[ 1/60  5/60 ]"  External=on  Measurements=None
  SwR2+ : powerlib/Elements/Breaker  BreakerResistance=Ron  InitialState=1  SnubberResistance=R  SnubberCapacitance=inf  SwitchingTimes="[ 1/60  5/60 ]"  External=on  Measurements=None
  SwR2- : powerlib/Elements/Breaker  BreakerResistance=Ron  InitialState=1  SnubberResistance=R  SnubberCapacitance=inf  SwitchingTimes="[ 1/60  5/60 ]"  External=on  Measurements=None
  Sw20 : PMIOPort  Port=1  Side=Left
  Sw19 : PMIOPort  Port=2  Side=Left
  Sw18 : PMIOPort  Port=3  Side=Left
  Sw17 : PMIOPort  Port=4  Side=Left
  Sw16 : PMIOPort  Port=5  Side=Left
  Sw15 : PMIOPort  Port=6  Side=Left
  Sw14 : PMIOPort  Port=7  Side=Left
  Sw13 : PMIOPort  Port=8  Side=Left
  Sw12 : PMIOPort  Port=9  Side=Left
  Sw11 : PMIOPort  Port=10  Side=Left
  Sw10 : PMIOPort  Port=11  Side=Left
  "Sw9 " : PMIOPort  Port=12  Side=Left
  Sw8 : PMIOPort  Port=13  Side=Left
  Sw7 : PMIOPort  Port=14  Side=Left
  Sw6 : PMIOPort  Port=15  Side=Left
  Sw5 : PMIOPort  Port=16  Side=Left
  Sw4 : PMIOPort  Port=17  Side=Left
  Sw3 : PMIOPort  Port=18  Side=Left
  "Sw2 " : PMIOPort  Port=19  Side=Left
  Sw1 : PMIOPort  Port=20  Side=Left
  Sw0 : PMIOPort  Port=21  Side=Left
  Out+ : PMIOPort  Orientation=left  Port=22  Side=Right
  Out- : PMIOPort  Orientation=left  Port=23  Side=Right
  wires:
  SwR/1 -> SwR2-/1, SwR1-/1, SwR1+/1, SwR2+/1
  Demux/6 -> 5/1
  Demux/7 -> 6/1
  Demux/8 -> 7/1
  Demux/9 -> 8/1
  Demux/10 -> 9/1
  Demux/11 -> 10-/1, "10+  "/1
  Demux/12 -> 11/1
  Demux/13 -> 12/1
  Demux/14 -> 13/1
  Demux/15 -> 14/1
  Demux/16 -> 15/1
  Demux/17 -> "16  "/1
  Demux/18 -> 17/1
  Demux/19 -> 18/1
  Demux/20 -> 19/1
  Demux/21 -> 20/1
  SwInv/1 -> Inversion/1(Inv)
  Demux/5 -> "4  "/1
  Demux/4 -> "3  "/1
  Demux/3 -> "2    "/1
  Demux/2 -> "1  "/1
  Demux/1 -> "0  "/1
  Sw0/10/1 -> Demux/1
  connections:
  Inversion/LConn1 -- SwR1+/RConn1 -- SwR2+/RConn1
  Sw10/RConn1 -- "10+  "/LConn1 -- 10-/LConn1
  SwR2+/LConn1 -- 19/RConn1 -- 17/RConn1 -- 15/RConn1 -- 13/RConn1 -- 11/RConn1
  SwR1+/LConn1 -- "10+  "/RConn1 -- 20/RConn1 -- 18/RConn1 -- "16  "/RConn1 -- 14/RConn1 -- 12/RConn1
  SwR2-/LConn1 -- "1  "/RConn1 -- "3  "/RConn1 -- 5/RConn1 -- 7/RConn1 -- 9/RConn1
  SwR1-/LConn1 -- "0  "/RConn1 -- "2    "/RConn1 -- "4  "/RConn1 -- 6/RConn1 -- 8/RConn1 -- 10-/RConn1
  Inversion/LConn2 -- SwR1-/RConn1 -- SwR2-/RConn1
  Sw11/RConn1 -- 11/LConn1
  Sw12/RConn1 -- 12/LConn1
  Sw13/RConn1 -- 13/LConn1
  Sw14/RConn1 -- 14/LConn1
  Sw15/RConn1 -- 15/LConn1
  "Sw9 "/RConn1 -- 9/LConn1
  Sw8/RConn1 -- 8/LConn1
  Sw7/RConn1 -- 7/LConn1
  Sw6/RConn1 -- 6/LConn1
  Sw5/RConn1 -- 5/LConn1
  Inversion/RConn2 -- Out-/RConn1
  Inversion/RConn1 -- Out+/RConn1
  Sw0/RConn1 -- "0  "/LConn1
  Sw1/RConn1 -- "1  "/LConn1
  "Sw2 "/RConn1 -- "2    "/LConn1
  Sw3/RConn1 -- "3  "/LConn1
  Sw4/RConn1 -- "4  "/LConn1
  Sw16/RConn1 -- "16  "/LConn1
  Sw17/RConn1 -- 17/LConn1
  Sw18/RConn1 -- 18/LConn1
  Sw19/RConn1 -- 19/LConn1
  Sw20/RConn1 -- 20/LConn1

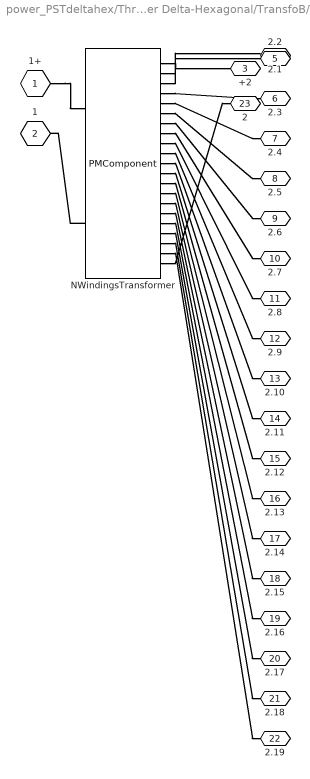
== system power_PSTdeltahex/Three-Phase OLTC Phase Shifting Transformer Delta-Hexagonal/TransfoB/Transformer ==
  NWindingsTransformer : PMComponent  PhysicalDomain=powersysdomain  LeftPortType=p1  RightPortType=p1  LConnTagsString=1|2  RConnTagsString=1|2|3|4|5|6|7|8|9|10|11|12|13|14|15|16|17|18|19|20|21
      mask Type: InnerPowersysBlock
  1+ : PMIOPort  Port=1  Side=Left
  1 : PMIOPort  Port=2  Side=Left
  +2 : PMIOPort  Orientation=left  Port=3  Side=Right
  2.1 : PMIOPort  Orientation=left  Port=4  Side=Right
  2.2 : PMIOPort  Orientation=left  Port=5  Side=Right
  2.3 : PMIOPort  Orientation=left  Port=6  Side=Right
  2.4 : PMIOPort  Orientation=left  Port=7  Side=Right
  2.5 : PMIOPort  Orientation=left  Port=8  Side=Right
  2.6 : PMIOPort  Orientation=left  Port=9  Side=Right
  2.7 : PMIOPort  Orientation=left  Port=10  Side=Right
  2.8 : PMIOPort  Orientation=left  Port=11  Side=Right
  2.9 : PMIOPort  Orientation=left  Port=12  Side=Right
  2.10 : PMIOPort  Orientation=left  Port=13  Side=Right
  2.11 : PMIOPort  Orientation=left  Port=14  Side=Right
  2.12 : PMIOPort  Orientation=left  Port=15  Side=Right
  2.13 : PMIOPort  Orientation=left  Port=16  Side=Right
  2.14 : PMIOPort  Orientation=left  Port=17  Side=Right
  2.15 : PMIOPort  Orientation=left  Port=18  Side=Right
  2.16 : PMIOPort  Orientation=left  Port=19  Side=Right
  2.17 : PMIOPort  Orientation=left  Port=20  Side=Right
  2.18 : PMIOPort  Orientation=left  Port=21  Side=Right
  2.19 : PMIOPort  Orientation=left  Port=22  Side=Right
  2 : PMIOPort  Orientation=left  Port=23  Side=Right
  connections:
  NWindingsTransformer/RConn20 -- 2.19/RConn1
  NWindingsTransformer/RConn19 -- 2.18/RConn1
  NWindingsTransformer/RConn18 -- 2.17/RConn1
  NWindingsTransformer/RConn17 -- 2.16/RConn1
  NWindingsTransformer/RConn16 -- 2.15/RConn1
  NWindingsTransformer/RConn15 -- 2.14/RConn1
  NWindingsTransformer/RConn14 -- 2.13/RConn1
  NWindingsTransformer/RConn13 -- 2.12/RConn1
  NWindingsTransformer/RConn12 -- 2.11/RConn1
  NWindingsTransformer/RConn11 -- 2.10/RConn1
  NWindingsTransformer/RConn21 -- 2/RConn1
  NWindingsTransformer/RConn10 -- 2.9/RConn1
  NWindingsTransformer/RConn9 -- 2.8/RConn1
  NWindingsTransformer/RConn8 -- 2.7/RConn1
  NWindingsTransformer/RConn7 -- 2.6/RConn1
  NWindingsTransformer/RConn6 -- 2.5/RConn1
  NWindingsTransformer/RConn5 -- 2.4/RConn1
  NWindingsTransformer/RConn4 -- 2.3/RConn1
  NWindingsTransformer/RConn3 -- 2.2/RConn1
  NWindingsTransformer/RConn2 -- 2.1/RConn1
  NWindingsTransformer/LConn2 -- 1/RConn1
  1+/RConn1 -- NWindingsTransformer/LConn1
  NWindingsTransformer/RConn1 -- +2/RConn1
